simulink model "MOBATSim"  (R2020a)
settings: Solver=VariableStepAuto  StartTime=0.0  StopTime=20  FixedStep=0.01  RelTol=1e-3
undefined symbols (not defined in the file): default_spacing, FI_distance, FI_speed, max_ac, meters, min_ac, SafeDistance, Sim_Ts, simSpeed, time_gap, Ts, v_set, Vehicle1, Vehicle10, Vehicle2, Vehicle3, Vehicle4, Vehicle5, Vehicle6, Vehicle7, Vehicle8, Vehicle9, verr_gain, vx_gain, xerr_gain
libraries: simulink x32, mpcadaslib x1, robotalgslib x1
(part 2 of 4)

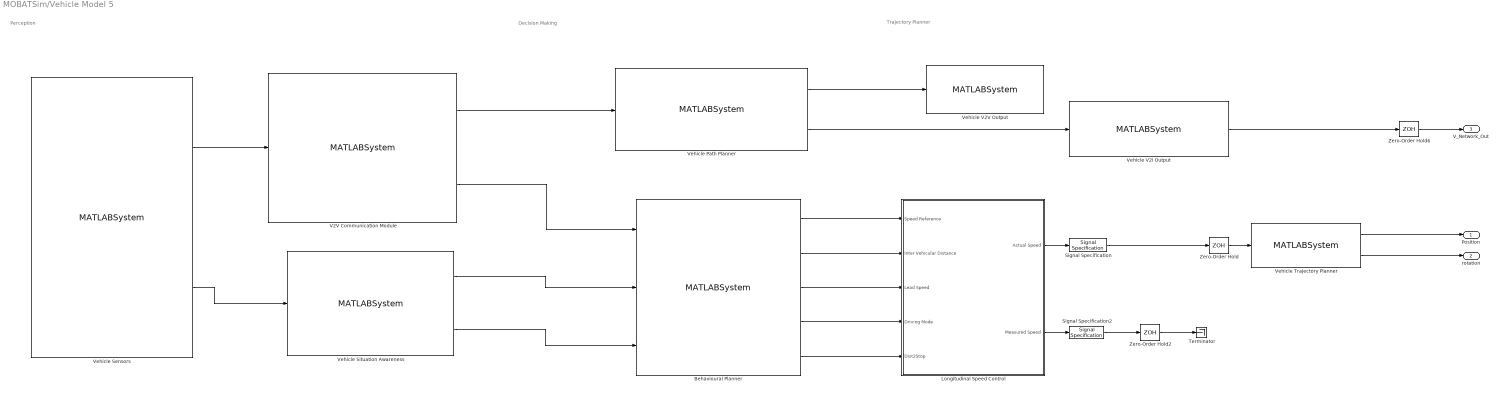
== system MOBATSim/Vehicle Model 5 ==
  note: Trajectory Planner
  note: Perception
  note: Decision Making
  Behavioural Planner : MATLABSystem  System=VehicleDrivingMode  Vehicle_id=Vehicle_id  SimulateUsing=Interpreted execution
      mask Type: VehicleDrivingMode
      mask Display:
      | image('BehaviouralPlanner.png');
      | port_label('input',1,'LeaderSpeed');
      | port_label('input',2,'LeaderDistance');
      | port_label('input',3,'emergencyCase');
      | port_label('output',1,'SpeedReference');
      | port_label('output',2,'DistanceReference');
      | port_label('output',3,'LeadSpeed');
      | port_label('output',4,'DrivingMode');
      | port_label('output',5,'Dist2Stop');
  Longitudinal Speed Control : Subsystem
  Signal Specification : SignalSpecification  Dimensions=1
  Signal Specification2 : SignalSpecification  Dimensions=1
  Terminator : Terminator
  V2V Communication Module : MATLABSystem  System=VehicleCommunication_v2v  Vehicle_id=Vehicle_id  SimulateUsing=Interpreted execution
      mask Type: VehicleCommunication_v2v
      mask Display:
      | image('V2V.png');
      | port_label('input',1,'CommunicationID');
      | port_label('output',1,'OtherVehiclesFutureData');
      | port_label('output',2,'LeaderSpeed');
  Vehicle Path Planner : MATLABSystem  System=VehiclePathPlanner  Vehicle_id=Vehicle_id  SimulateUsing=Interpreted execution
      mask Type: VehiclePathPlanner
      mask Display:
      | image('PathPlanner.png');
      | port_label('input',1,'OtherVehiclesFutureData');
      | port_label('output',1,'FuturePlan');
      | port_label('output',2,'waypointReached');
  Vehicle Sensors : MATLABSystem  System=VehicleSensors  Vehicle_id=Vehicle_id  Tsample=Sim_Ts  OffsetTime=0  SimulateUsing=Interpreted execution
      mask Type: VehicleSensors
      mask Display:
      | image('sensor.png');
      | port_label('output',1,'V2VcommIDs');
      | port_label('output',2,'ObjectinFront');
  Vehicle Situation Awareness : MATLABSystem  System=VehicleSituationAwareness  Vehicle_id=Vehicle_id  SimulateUsing=Interpreted execution
      mask Type: VehicleSituationAwareness
      mask Display:
      | image('situationAwareness.png');
      | port_label('input',1,'FrontSensorData');
      | port_label('output',1,'leaderDistance');
      | port_label('output',2,'emergencyCase');
  Vehicle Trajectory Planner : MATLABSystem  System=VehicleKinematics  Vehicle_id=Vehicle_id  SimulateUsing=Interpreted execution
      mask Type: VehicleKinematics
      mask Display:
      | image('Vehicle.png');
      | port_label('input',1,'speed');
      | port_label('output',1,'position');
      | port_label('output',2,'rotation');
  Vehicle V2I Output : MATLABSystem  System=VehicleV2I_Out  Vehicle_id=Vehicle_id  SimulateUsing=Interpreted execution
      mask Type: VehicleV2I_Out
      mask Display:
      | image('V2I.png');
      | port_label('input',1,'waypointReached');
      | port_label('output',1,'V2Idata');
  Vehicle V2V Output : MATLABSystem  System=VehicleNetwork_Out  Vehicle_id=Vehicle_id  SimulateUsing=Interpreted execution
      mask Type: VehicleNetwork_Out
      mask Display:
      | image('V2V.png');
      | port_label('input',1,'FuturePlan');
  Zero-Order Hold : ZeroOrderHold  SampleTime=Sim_Ts
  Zero-Order Hold2 : ZeroOrderHold  SampleTime=Sim_Ts
  Zero-Order Hold6 : ZeroOrderHold  SampleTime=Sim_Ts
  Position : Outport  VectorParamsAs1DForOutWhenUnconnected=off
  rotation : Outport  Port=2  VectorParamsAs1DForOutWhenUnconnected=off
  V_Network_Out : Outport  Port=3  VectorParamsAs1DForOutWhenUnconnected=off
  wires:
  Vehicle Trajectory Planner/1 -> Position/1
  Vehicle Trajectory Planner/2 -> rotation/1
  Signal Specification/1 -> Zero-Order Hold/1
  Zero-Order Hold/1 -> Vehicle Trajectory Planner/1
  Signal Specification2/1 -> Zero-Order Hold2/1
  Longitudinal Speed Control/1(Actual Speed) -> Signal Specification/1
  Vehicle V2I Output/1 -> Zero-Order Hold6/1
  Longitudinal Speed Control/2(Measured Speed) -> Signal Specification2/1
  Zero-Order Hold2/1 -> Terminator/1
  Vehicle Sensors/2 -> Vehicle Situation Awareness/1
  Vehicle Situation Awareness/2 -> Behavioural Planner/3
  Vehicle Situation Awareness/1 -> Behavioural Planner/2
  V2V Communication Module/2 -> Behavioural Planner/1
  V2V Communication Module/1 -> Vehicle Path Planner/1
  Behavioural Planner/5 -> Longitudinal Speed Control/5(Dist2Stop)
  Behavioural Planner/4 -> Longitudinal Speed Control/4(Driving Mode)
  Behavioural Planner/3 -> Longitudinal Speed Control/3(Lead Speed)
  Behavioural Planner/2 -> Longitudinal Speed Control/2(Inter Vehicular Distance)
  Behavioural Planner/1 -> Longitudinal Speed Control/1(Speed Reference)
  Vehicle Path Planner/2 -> Vehicle V2I Output/1
  Vehicle Path Planner/1 -> Vehicle V2V Output/1
  Vehicle Sensors/1 -> V2V Communication Module/1
  Zero-Order Hold6/1 -> V_Network_Out/1

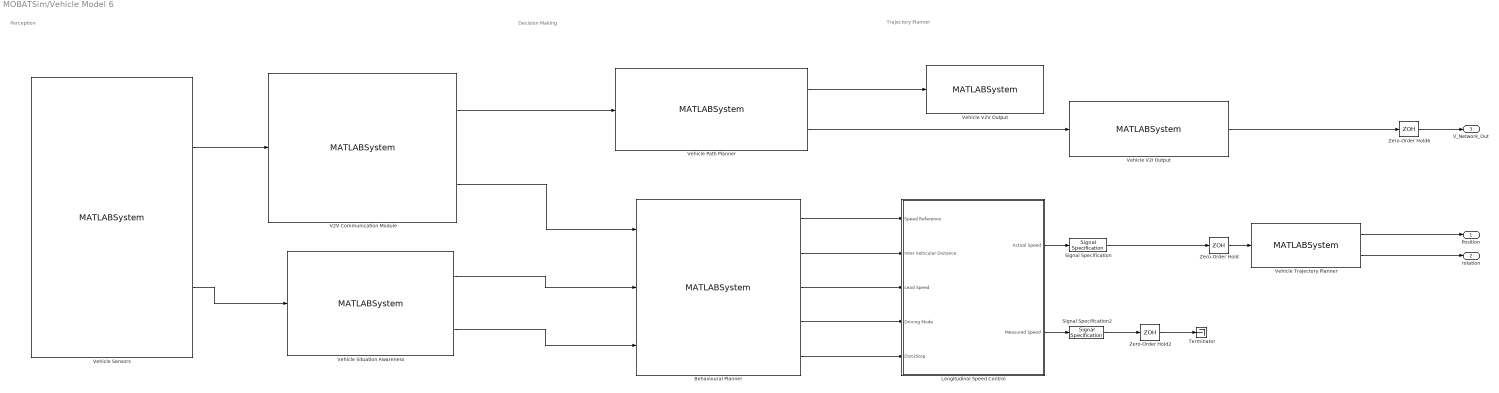
== system MOBATSim/Vehicle Model 6 ==
  note: Trajectory Planner
  note: Perception
  note: Decision Making
  Behavioural Planner : MATLABSystem  System=VehicleDrivingMode  Vehicle_id=Vehicle_id  SimulateUsing=Interpreted execution
      mask Type: VehicleDrivingMode
      mask Display:
      | image('BehaviouralPlanner.png');
      | port_label('input',1,'LeaderSpeed');
      | port_label('input',2,'LeaderDistance');
      | port_label('input',3,'emergencyCase');
      | port_label('output',1,'SpeedReference');
      | port_label('output',2,'DistanceReference');
      | port_label('output',3,'LeadSpeed');
      | port_label('output',4,'DrivingMode');
      | port_label('output',5,'Dist2Stop');
  Longitudinal Speed Control : Subsystem
  Signal Specification : SignalSpecification  Dimensions=1
  Signal Specification2 : SignalSpecification  Dimensions=1
  Terminator : Terminator
  V2V Communication Module : MATLABSystem  System=VehicleCommunication_v2v  Vehicle_id=Vehicle_id  SimulateUsing=Interpreted execution
      mask Type: VehicleCommunication_v2v
      mask Display:
      | image('V2V.png');
      | port_label('input',1,'CommunicationID');
      | port_label('output',1,'OtherVehiclesFutureData');
      | port_label('output',2,'LeaderSpeed');
  Vehicle Path Planner : MATLABSystem  System=VehiclePathPlanner  Vehicle_id=Vehicle_id  SimulateUsing=Interpreted execution
      mask Type: VehiclePathPlanner
      mask Display:
      | image('PathPlanner.png');
      | port_label('input',1,'OtherVehiclesFutureData');
      | port_label('output',1,'FuturePlan');
      | port_label('output',2,'waypointReached');
  Vehicle Sensors : MATLABSystem  System=VehicleSensors  Vehicle_id=Vehicle_id  Tsample=Sim_Ts  OffsetTime=0  SimulateUsing=Interpreted execution
      mask Type: VehicleSensors
      mask Display:
      | image('sensor.png');
      | port_label('output',1,'V2VcommIDs');
      | port_label('output',2,'ObjectinFront');
  Vehicle Situation Awareness : MATLABSystem  System=VehicleSituationAwareness  Vehicle_id=Vehicle_id  SimulateUsing=Interpreted execution
      mask Type: VehicleSituationAwareness
      mask Display:
      | image('situationAwareness.png');
      | port_label('input',1,'FrontSensorData');
      | port_label('output',1,'leaderDistance');
      | port_label('output',2,'emergencyCase');
  Vehicle Trajectory Planner : MATLABSystem  System=VehicleKinematics  Vehicle_id=Vehicle_id  SimulateUsing=Interpreted execution
      mask Type: VehicleKinematics
      mask Display:
      | image('Vehicle.png');
      | port_label('input',1,'speed');
      | port_label('output',1,'position');
      | port_label('output',2,'rotation');
  Vehicle V2I Output : MATLABSystem  System=VehicleV2I_Out  Vehicle_id=Vehicle_id  SimulateUsing=Interpreted execution
      mask Type: VehicleV2I_Out
      mask Display:
      | image('V2I.png');
      | port_label('input',1,'waypointReached');
      | port_label('output',1,'V2Idata');
  Vehicle V2V Output : MATLABSystem  System=VehicleNetwork_Out  Vehicle_id=Vehicle_id  SimulateUsing=Interpreted execution
      mask Type: VehicleNetwork_Out
      mask Display:
      | image('V2V.png');
      | port_label('input',1,'FuturePlan');
  Zero-Order Hold : ZeroOrderHold  SampleTime=Sim_Ts
  Zero-Order Hold2 : ZeroOrderHold  SampleTime=Sim_Ts
  Zero-Order Hold6 : ZeroOrderHold  SampleTime=Sim_Ts
  Position : Outport  VectorParamsAs1DForOutWhenUnconnected=off
  rotation : Outport  Port=2  VectorParamsAs1DForOutWhenUnconnected=off
  V_Network_Out : Outport  Port=3  VectorParamsAs1DForOutWhenUnconnected=off
  wires:
  Vehicle Trajectory Planner/1 -> Position/1
  Vehicle Trajectory Planner/2 -> rotation/1
  Signal Specification/1 -> Zero-Order Hold/1
  Zero-Order Hold/1 -> Vehicle Trajectory Planner/1
  Signal Specification2/1 -> Zero-Order Hold2/1
  Longitudinal Speed Control/1(Actual Speed) -> Signal Specification/1
  Vehicle V2I Output/1 -> Zero-Order Hold6/1
  Longitudinal Speed Control/2(Measured Speed) -> Signal Specification2/1
  Zero-Order Hold2/1 -> Terminator/1
  Vehicle Sensors/2 -> Vehicle Situation Awareness/1
  Vehicle Situation Awareness/2 -> Behavioural Planner/3
  Vehicle Situation Awareness/1 -> Behavioural Planner/2
  V2V Communication Module/2 -> Behavioural Planner/1
  V2V Communication Module/1 -> Vehicle Path Planner/1
  Behavioural Planner/5 -> Longitudinal Speed Control/5(Dist2Stop)
  Behavioural Planner/4 -> Longitudinal Speed Control/4(Driving Mode)
  Behavioural Planner/3 -> Longitudinal Speed Control/3(Lead Speed)
  Behavioural Planner/2 -> Longitudinal Speed Control/2(Inter Vehicular Distance)
  Behavioural Planner/1 -> Longitudinal Speed Control/1(Speed Reference)
  Vehicle Path Planner/2 -> Vehicle V2I Output/1
  Vehicle Path Planner/1 -> Vehicle V2V Output/1
  Vehicle Sensors/1 -> V2V Communication Module/1
  Zero-Order Hold6/1 -> V_Network_Out/1

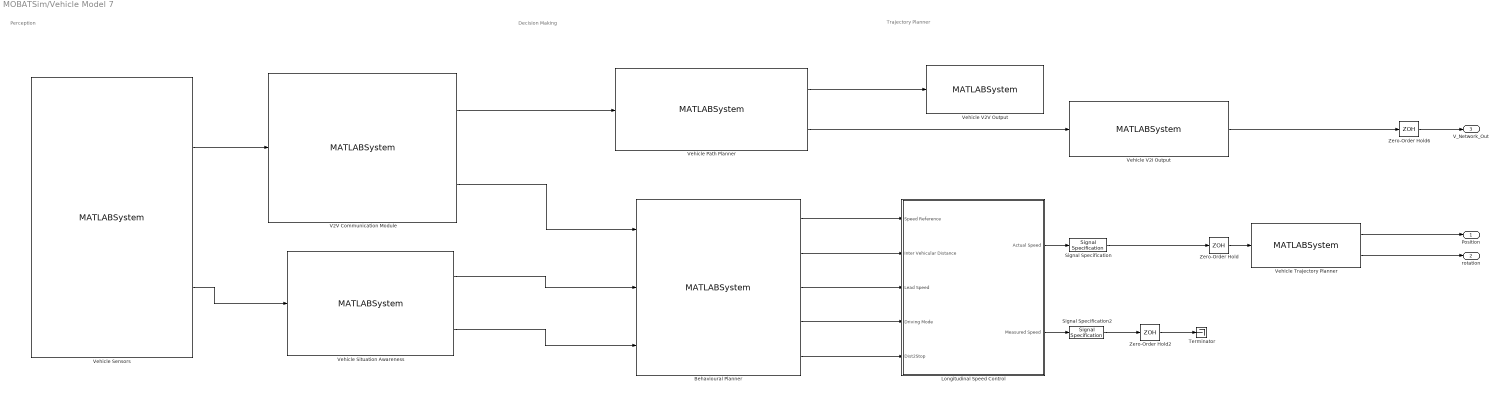
== system MOBATSim/Vehicle Model 7 ==
  note: Trajectory Planner
  note: Perception
  note: Decision Making
  Behavioural Planner : MATLABSystem  System=VehicleDrivingMode  Vehicle_id=Vehicle_id  SimulateUsing=Interpreted execution
      mask Type: VehicleDrivingMode
      mask Display:
      | image('BehaviouralPlanner.png');
      | port_label('input',1,'LeaderSpeed');
      | port_label('input',2,'LeaderDistance');
      | port_label('input',3,'emergencyCase');
      | port_label('output',1,'SpeedReference');
      | port_label('output',2,'DistanceReference');
      | port_label('output',3,'LeadSpeed');
      | port_label('output',4,'DrivingMode');
      | port_label('output',5,'Dist2Stop');
  Longitudinal Speed Control : Subsystem
  Signal Specification : SignalSpecification  Dimensions=1
  Signal Specification2 : SignalSpecification  Dimensions=1
  Terminator : Terminator
  V2V Communication Module : MATLABSystem  System=VehicleCommunication_v2v  Vehicle_id=Vehicle_id  SimulateUsing=Interpreted execution
      mask Type: VehicleCommunication_v2v
      mask Display:
      | image('V2V.png');
      | port_label('input',1,'CommunicationID');
      | port_label('output',1,'OtherVehiclesFutureData');
      | port_label('output',2,'LeaderSpeed');
  Vehicle Path Planner : MATLABSystem  System=VehiclePathPlanner  Vehicle_id=Vehicle_id  SimulateUsing=Interpreted execution
      mask Type: VehiclePathPlanner
      mask Display:
      | image('PathPlanner.png');
      | port_label('input',1,'OtherVehiclesFutureData');
      | port_label('output',1,'FuturePlan');
      | port_label('output',2,'waypointReached');
  Vehicle Sensors : MATLABSystem  System=VehicleSensors  Vehicle_id=Vehicle_id  Tsample=Sim_Ts  OffsetTime=0  SimulateUsing=Interpreted execution
      mask Type: VehicleSensors
      mask Display:
      | image('sensor.png');
      | port_label('output',1,'V2VcommIDs');
      | port_label('output',2,'ObjectinFront');
  Vehicle Situation Awareness : MATLABSystem  System=VehicleSituationAwareness  Vehicle_id=Vehicle_id  SimulateUsing=Interpreted execution
      mask Type: VehicleSituationAwareness
      mask Display:
      | image('situationAwareness.png');
      | port_label('input',1,'FrontSensorData');
      | port_label('output',1,'leaderDistance');
      | port_label('output',2,'emergencyCase');
  Vehicle Trajectory Planner : MATLABSystem  System=VehicleKinematics  Vehicle_id=Vehicle_id  SimulateUsing=Interpreted execution
      mask Type: VehicleKinematics
      mask Display:
      | image('Vehicle.png');
      | port_label('input',1,'speed');
      | port_label('output',1,'position');
      | port_label('output',2,'rotation');
  Vehicle V2I Output : MATLABSystem  System=VehicleV2I_Out  Vehicle_id=Vehicle_id  SimulateUsing=Interpreted execution
      mask Type: VehicleV2I_Out
      mask Display:
      | image('V2I.png');
      | port_label('input',1,'waypointReached');
      | port_label('output',1,'V2Idata');
  Vehicle V2V Output : MATLABSystem  System=VehicleNetwork_Out  Vehicle_id=Vehicle_id  SimulateUsing=Interpreted execution
      mask Type: VehicleNetwork_Out
      mask Display:
      | image('V2V.png');
      | port_label('input',1,'FuturePlan');
  Zero-Order Hold : ZeroOrderHold  SampleTime=Sim_Ts
  Zero-Order Hold2 : ZeroOrderHold  SampleTime=Sim_Ts
  Zero-Order Hold6 : ZeroOrderHold  SampleTime=Sim_Ts
  Position : Outport  VectorParamsAs1DForOutWhenUnconnected=off
  rotation : Outport  Port=2  VectorParamsAs1DForOutWhenUnconnected=off
  V_Network_Out : Outport  Port=3  VectorParamsAs1DForOutWhenUnconnected=off
  wires:
  Vehicle Trajectory Planner/1 -> Position/1
  Vehicle Trajectory Planner/2 -> rotation/1
  Signal Specification/1 -> Zero-Order Hold/1
  Zero-Order Hold/1 -> Vehicle Trajectory Planner/1
  Signal Specification2/1 -> Zero-Order Hold2/1
  Longitudinal Speed Control/1(Actual Speed) -> Signal Specification/1
  Vehicle V2I Output/1 -> Zero-Order Hold6/1
  Longitudinal Speed Control/2(Measured Speed) -> Signal Specification2/1
  Zero-Order Hold2/1 -> Terminator/1
  Vehicle Sensors/2 -> Vehicle Situation Awareness/1
  Vehicle Situation Awareness/2 -> Behavioural Planner/3
  Vehicle Situation Awareness/1 -> Behavioural Planner/2
  V2V Communication Module/2 -> Behavioural Planner/1
  V2V Communication Module/1 -> Vehicle Path Planner/1
  Behavioural Planner/5 -> Longitudinal Speed Control/5(Dist2Stop)
  Behavioural Planner/4 -> Longitudinal Speed Control/4(Driving Mode)
  Behavioural Planner/3 -> Longitudinal Speed Control/3(Lead Speed)
  Behavioural Planner/2 -> Longitudinal Speed Control/2(Inter Vehicular Distance)
  Behavioural Planner/1 -> Longitudinal Speed Control/1(Speed Reference)
  Vehicle Path Planner/2 -> Vehicle V2I Output/1
  Vehicle Path Planner/1 -> Vehicle V2V Output/1
  Vehicle Sensors/1 -> V2V Communication Module/1
  Zero-Order Hold6/1 -> V_Network_Out/1

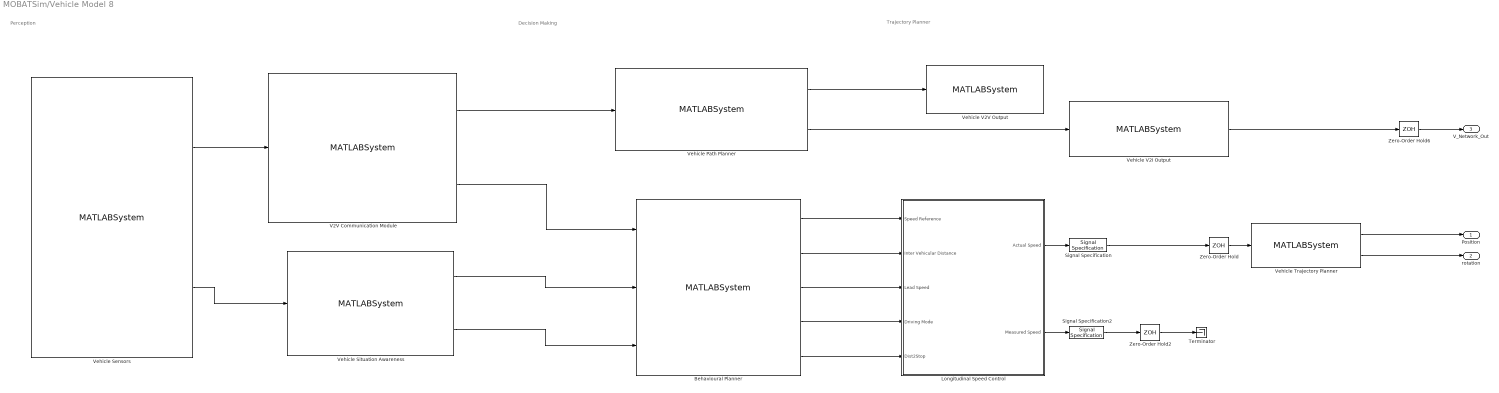
== system MOBATSim/Vehicle Model 8 ==
  note: Trajectory Planner
  note: Perception
  note: Decision Making
  Behavioural Planner : MATLABSystem  System=VehicleDrivingMode  Vehicle_id=Vehicle_id  SimulateUsing=Interpreted execution
      mask Type: VehicleDrivingMode
      mask Display:
      | image('BehaviouralPlanner.png');
      | port_label('input',1,'LeaderSpeed');
      | port_label('input',2,'LeaderDistance');
      | port_label('input',3,'emergencyCase');
      | port_label('output',1,'SpeedReference');
      | port_label('output',2,'DistanceReference');
      | port_label('output',3,'LeadSpeed');
      | port_label('output',4,'DrivingMode');
      | port_label('output',5,'Dist2Stop');
  Longitudinal Speed Control : Subsystem
  Signal Specification : SignalSpecification  Dimensions=1
  Signal Specification2 : SignalSpecification  Dimensions=1
  Terminator : Terminator
  V2V Communication Module : MATLABSystem  System=VehicleCommunication_v2v  Vehicle_id=Vehicle_id  SimulateUsing=Interpreted execution
      mask Type: VehicleCommunication_v2v
      mask Display:
      | image('V2V.png');
      | port_label('input',1,'CommunicationID');
      | port_label('output',1,'OtherVehiclesFutureData');
      | port_label('output',2,'LeaderSpeed');
  Vehicle Path Planner : MATLABSystem  System=VehiclePathPlanner  Vehicle_id=Vehicle_id  SimulateUsing=Interpreted execution
      mask Type: VehiclePathPlanner
      mask Display:
      | image('PathPlanner.png');
      | port_label('input',1,'OtherVehiclesFutureData');
      | port_label('output',1,'FuturePlan');
      | port_label('output',2,'waypointReached');
  Vehicle Sensors : MATLABSystem  System=VehicleSensors  Vehicle_id=Vehicle_id  Tsample=Sim_Ts  OffsetTime=0  SimulateUsing=Interpreted execution
      mask Type: VehicleSensors
      mask Display:
      | image('sensor.png');
      | port_label('output',1,'V2VcommIDs');
      | port_label('output',2,'ObjectinFront');
  Vehicle Situation Awareness : MATLABSystem  System=VehicleSituationAwareness  Vehicle_id=Vehicle_id  SimulateUsing=Interpreted execution
      mask Type: VehicleSituationAwareness
      mask Display:
      | image('situationAwareness.png');
      | port_label('input',1,'FrontSensorData');
      | port_label('output',1,'leaderDistance');
      | port_label('output',2,'emergencyCase');
  Vehicle Trajectory Planner : MATLABSystem  System=VehicleKinematics  Vehicle_id=Vehicle_id  SimulateUsing=Interpreted execution
      mask Type: VehicleKinematics
      mask Display:
      | image('Vehicle.png');
      | port_label('input',1,'speed');
      | port_label('output',1,'position');
      | port_label('output',2,'rotation');
  Vehicle V2I Output : MATLABSystem  System=VehicleV2I_Out  Vehicle_id=Vehicle_id  SimulateUsing=Interpreted execution
      mask Type: VehicleV2I_Out
      mask Display:
      | image('V2I.png');
      | port_label('input',1,'waypointReached');
      | port_label('output',1,'V2Idata');
  Vehicle V2V Output : MATLABSystem  System=VehicleNetwork_Out  Vehicle_id=Vehicle_id  SimulateUsing=Interpreted execution
      mask Type: VehicleNetwork_Out
      mask Display:
      | image('V2V.png');
      | port_label('input',1,'FuturePlan');
  Zero-Order Hold : ZeroOrderHold  SampleTime=Sim_Ts
  Zero-Order Hold2 : ZeroOrderHold  SampleTime=Sim_Ts
  Zero-Order Hold6 : ZeroOrderHold  SampleTime=Sim_Ts
  Position : Outport  VectorParamsAs1DForOutWhenUnconnected=off
  rotation : Outport  Port=2  VectorParamsAs1DForOutWhenUnconnected=off
  V_Network_Out : Outport  Port=3  VectorParamsAs1DForOutWhenUnconnected=off
  wires:
  Vehicle Trajectory Planner/1 -> Position/1
  Vehicle Trajectory Planner/2 -> rotation/1
  Signal Specification/1 -> Zero-Order Hold/1
  Zero-Order Hold/1 -> Vehicle Trajectory Planner/1
  Signal Specification2/1 -> Zero-Order Hold2/1
  Longitudinal Speed Control/1(Actual Speed) -> Signal Specification/1
  Vehicle V2I Output/1 -> Zero-Order Hold6/1
  Longitudinal Speed Control/2(Measured Speed) -> Signal Specification2/1
  Zero-Order Hold2/1 -> Terminator/1
  Vehicle Sensors/2 -> Vehicle Situation Awareness/1
  Vehicle Situation Awareness/2 -> Behavioural Planner/3
  Vehicle Situation Awareness/1 -> Behavioural Planner/2
  V2V Communication Module/2 -> Behavioural Planner/1
  V2V Communication Module/1 -> Vehicle Path Planner/1
  Behavioural Planner/5 -> Longitudinal Speed Control/5(Dist2Stop)
  Behavioural Planner/4 -> Longitudinal Speed Control/4(Driving Mode)
  Behavioural Planner/3 -> Longitudinal Speed Control/3(Lead Speed)
  Behavioural Planner/2 -> Longitudinal Speed Control/2(Inter Vehicular Distance)
  Behavioural Planner/1 -> Longitudinal Speed Control/1(Speed Reference)
  Vehicle Path Planner/2 -> Vehicle V2I Output/1
  Vehicle Path Planner/1 -> Vehicle V2V Output/1
  Vehicle Sensors/1 -> V2V Communication Module/1
  Zero-Order Hold6/1 -> V_Network_Out/1

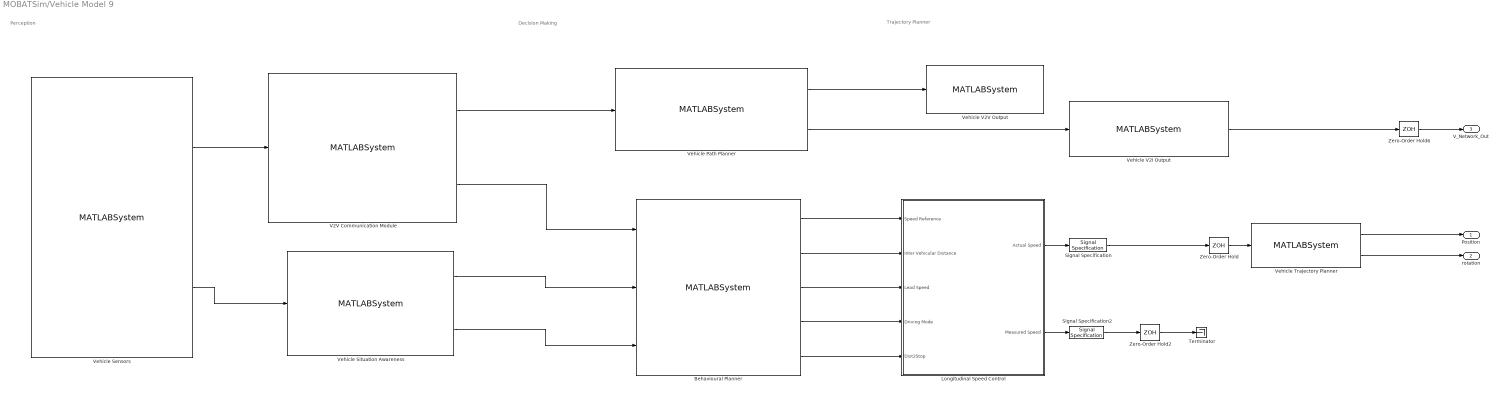
== system MOBATSim/Vehicle Model 9 ==
  note: Trajectory Planner
  note: Perception
  note: Decision Making
  Behavioural Planner : MATLABSystem  System=VehicleDrivingMode  Vehicle_id=Vehicle_id  SimulateUsing=Interpreted execution
      mask Type: VehicleDrivingMode
      mask Display:
      | image('BehaviouralPlanner.png');
      | port_label('input',1,'LeaderSpeed');
      | port_label('input',2,'LeaderDistance');
      | port_label('input',3,'emergencyCase');
      | port_label('output',1,'SpeedReference');
      | port_label('output',2,'DistanceReference');
      | port_label('output',3,'LeadSpeed');
      | port_label('output',4,'DrivingMode');
      | port_label('output',5,'Dist2Stop');
  Longitudinal Speed Control : Subsystem
  Signal Specification : SignalSpecification  Dimensions=1
  Signal Specification2 : SignalSpecification  Dimensions=1
  Terminator : Terminator
  V2V Communication Module : MATLABSystem  System=VehicleCommunication_v2v  Vehicle_id=Vehicle_id  SimulateUsing=Interpreted execution
      mask Type: VehicleCommunication_v2v
      mask Display:
      | image('V2V.png');
      | port_label('input',1,'CommunicationID');
      | port_label('output',1,'OtherVehiclesFutureData');
      | port_label('output',2,'LeaderSpeed');
  Vehicle Path Planner : MATLABSystem  System=VehiclePathPlanner  Vehicle_id=Vehicle_id  SimulateUsing=Interpreted execution
      mask Type: VehiclePathPlanner
      mask Display:
      | image('PathPlanner.png');
      | port_label('input',1,'OtherVehiclesFutureData');
      | port_label('output',1,'FuturePlan');
      | port_label('output',2,'waypointReached');
  Vehicle Sensors : MATLABSystem  System=VehicleSensors  Vehicle_id=Vehicle_id  Tsample=Sim_Ts  OffsetTime=0  SimulateUsing=Interpreted execution
      mask Type: VehicleSensors
      mask Display:
      | image('sensor.png');
      | port_label('output',1,'V2VcommIDs');
      | port_label('output',2,'ObjectinFront');
  Vehicle Situation Awareness : MATLABSystem  System=VehicleSituationAwareness  Vehicle_id=Vehicle_id  SimulateUsing=Interpreted execution
      mask Type: VehicleSituationAwareness
      mask Display:
      | image('situationAwareness.png');
      | port_label('input',1,'FrontSensorData');
      | port_label('output',1,'leaderDistance');
      | port_label('output',2,'emergencyCase');
  Vehicle Trajectory Planner : MATLABSystem  System=VehicleKinematics  Vehicle_id=Vehicle_id  SimulateUsing=Interpreted execution
      mask Type: VehicleKinematics
      mask Display:
      | image('Vehicle.png');
      | port_label('input',1,'speed');
      | port_label('output',1,'position');
      | port_label('output',2,'rotation');
  Vehicle V2I Output : MATLABSystem  System=VehicleV2I_Out  Vehicle_id=Vehicle_id  SimulateUsing=Interpreted execution
      mask Type: VehicleV2I_Out
      mask Display:
      | image('V2I.png');
      | port_label('input',1,'waypointReached');
      | port_label('output',1,'V2Idata');
  Vehicle V2V Output : MATLABSystem  System=VehicleNetwork_Out  Vehicle_id=Vehicle_id  SimulateUsing=Interpreted execution
      mask Type: VehicleNetwork_Out
      mask Display:
      | image('V2V.png');
      | port_label('input',1,'FuturePlan');
  Zero-Order Hold : ZeroOrderHold  SampleTime=Sim_Ts
  Zero-Order Hold2 : ZeroOrderHold  SampleTime=Sim_Ts
  Zero-Order Hold6 : ZeroOrderHold  SampleTime=Sim_Ts
  Position : Outport  VectorParamsAs1DForOutWhenUnconnected=off
  rotation : Outport  Port=2  VectorParamsAs1DForOutWhenUnconnected=off
  V_Network_Out : Outport  Port=3  VectorParamsAs1DForOutWhenUnconnected=off
  wires:
  Vehicle Trajectory Planner/1 -> Position/1
  Vehicle Trajectory Planner/2 -> rotation/1
  Signal Specification/1 -> Zero-Order Hold/1
  Zero-Order Hold/1 -> Vehicle Trajectory Planner/1
  Signal Specification2/1 -> Zero-Order Hold2/1
  Longitudinal Speed Control/1(Actual Speed) -> Signal Specification/1
  Vehicle V2I Output/1 -> Zero-Order Hold6/1
  Longitudinal Speed Control/2(Measured Speed) -> Signal Specification2/1
  Zero-Order Hold2/1 -> Terminator/1
  Vehicle Sensors/2 -> Vehicle Situation Awareness/1
  Vehicle Situation Awareness/2 -> Behavioural Planner/3
  Vehicle Situation Awareness/1 -> Behavioural Planner/2
  V2V Communication Module/2 -> Behavioural Planner/1
  V2V Communication Module/1 -> Vehicle Path Planner/1
  Behavioural Planner/5 -> Longitudinal Speed Control/5(Dist2Stop)
  Behavioural Planner/4 -> Longitudinal Speed Control/4(Driving Mode)
  Behavioural Planner/3 -> Longitudinal Speed Control/3(Lead Speed)
  Behavioural Planner/2 -> Longitudinal Speed Control/2(Inter Vehicular Distance)
  Behavioural Planner/1 -> Longitudinal Speed Control/1(Speed Reference)
  Vehicle Path Planner/2 -> Vehicle V2I Output/1
  Vehicle Path Planner/1 -> Vehicle V2V Output/1
  Vehicle Sensors/1 -> V2V Communication Module/1
  Zero-Order Hold6/1 -> V_Network_Out/1

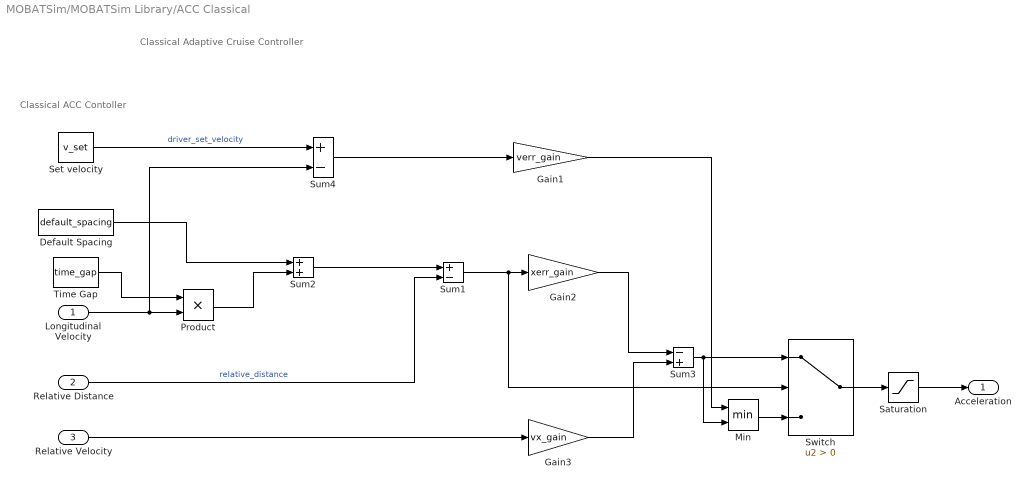
== system MOBATSim/MOBATSim Library/ACC Classical ==
  note: Classical ACC Contoller
  note: Classical Adaptive Cruise Controller
  Longitudinal Velocity : Inport
  Relative Distance : Inport  Port=2
  Relative Velocity : Inport  Port=3
  Default Spacing : Constant  Value=default_spacing  SampleTime=Ts
  Gain1 : Gain  Gain=verr_gain
  Gain2 : Gain  Gain=xerr_gain
  Gain3 : Gain  Gain=vx_gain
  Min : MinMax  Inputs=2
  Product : Product
  Saturation : Saturate  UpperLimit=max_ac  LowerLimit=min_ac
  Set velocity : Constant  Value=v_set  SampleTime=Ts
  Sum1 : Sum  Inputs=+-
  Sum2 : Sum
  Sum3 : Sum  Inputs=-+
  Sum4 : Sum  Inputs=+-
  Switch : Switch  Criteria=u2 > Threshold
  Time Gap : Constant  Value=time_gap  SampleTime=Ts
  Acceleration : Outport  VectorParamsAs1DForOutWhenUnconnected=off
  wires:
  Longitudinal Velocity/1 -> Product/2, Sum4/2
  Default Spacing/1 -> Sum2/1
  Gain2/1 -> Sum3/1
  Sum4/1 -> Gain1/1
  Min/1 -> Switch/3
  Gain3/1 -> Sum3/2
  Switch/1 -> Saturation/1
  Relative Velocity/1 -> Gain3/1
  Time Gap/1 -> Product/1
  Saturation/1 -> Acceleration/1
  Product/1 -> Sum2/2
  Set velocity/1 -> Sum4/1  "driver_set_velocity"
  Sum3/1 -> Min/2, Switch/1
  Sum1/1 -> Switch/2, Gain2/1
  Gain1/1 -> Min/1
  Relative Distance/1 -> Sum1/2  "relative_distance"
  Sum2/1 -> Sum1/1

== system MOBATSim/MOBATSim Library/Platoon Controller - PID ==
  Inter Vehicular Distance : Inport
  Lead Speed : Inport  Port=2
  Vehicle Speed : Inport  Port=3
  Compare To Constant : simulink/Logic and Bit Operations/Compare To Constant  relop=>  const=2  OutDataTypeStr=uint8
  Constant : Constant  Value=meters
  Gain : Gain  Gain=1.4
  Multiport Switch : MultiPortSwitch  DataPortOrder=Zero-based contiguous  Inputs=2  zeroidx=on
  PID Controller5 : simulink/Continuous/PID Controller  Controller=PID  Form=Parallel  TimeDomain=Continuous-time  UseExternalTs=off  SampleTime=-1  IntegratorMethod=Forward Euler  FilterMethod=Forward Euler  ControllerParametersSource=internal  P=2.0341199375219  I=0.0356576460366845  D=2.08363010404189  UseFilter=on  N=233.214579742572  TunerSelectOption=Transfer Function Based (PID Tuner App)  InitialConditionSource=internal  InitialConditionForIntegrator=0  InitialConditionForFilter=0  DifferentiatorICPrevScaledInput=0  ExternalReset=none  TrackingMode=off  Kt=1  LimitOutput=on  UpperSaturationLimit=100  LowerSaturationLimit=-100  LinearizeAsGain=on  AntiWindupMode=clamping  Kb=1  POutMin=[]  POutMax=[]  IOutMin=[]  IOutMax=[]  DOutMin=[]  DOutMax=[]  NOutMin=[]  NOutMax=[]  SumOutMin=[]  SumOutMax=[]  SaturationOutMin=[]  SaturationOutMax=[]  PParamMin=[]  PParamMax=[]  IParamMin=[]  IParamMax=[]  DParamMin=[]  DParamMax=[]  NParamMin=[]  NParamMax=[]  KbParamMin=[]  KbParamMax=[]  KtParamMin=[]  KtParamMax=[]  KbOutMin=[]  KbOutMax=[]  KtOutMin=[]  KtOutMax=[]  IntegratorOutMin=[]  IntegratorOutMax=[]  FilterOutMin=[]  FilterOutMax=[]  SumI1OutMin=[]  SumI1OutMax=[]  SumI2OutMin=[]  SumI2OutMax=[]  SumI3OutMin=[]  SumI3OutMax=[]  SumI4OutMin=[]  SumI4OutMax=[]  SumDOutMin=[]  SumDOutMax=[]  DifferentiatorOutMin=[]  DifferentiatorOutMax=[]  FilterDiffOutCoefMin=[]  FilterDiffOutCoefMax=[]  ReciprocalOutMin=[]  ReciprocalOutMax=[]  SumDenOutMin=[]  SumDenOutMax=[]  SumNumOutMin=[]  SumNumOutMax=[]  DivideOutMin=[]  DivideOutMax=[]  UdiffTsProdOutMin=[]  UdiffTsProdOutMax=[]  NTsProdOutMin=[]  NTsProdOutMax=[]  UintegralTsProdOutMin=[]  UintegralTsProdOutMax=[]  UngainTsProdOutMin=[]  UngainTsProdOutMax=[]  IntegratorContinuousStateAttributes=''  IntegratorStateMustResolveToSignalObject=off  IntegratorRTWStateStorageClass=Auto  FilterContinuousStateAttributes=''  FilterStateMustResolveToSignalObject=off  FilterRTWStateStorageClass=Auto  ParallelPVariant=InternalParameters  IdealPVariant=Disabled  IVariant=InternalParameters  DVariant=InternalParameters  IntegratorVariant=Continuous  SatVariant=Enabled  AWVariant=ContClampingParallel  PCopyVariant=Disabled  TRVariant=Disabled  FdbkBlocksVariant=Forward  IdealPFdbkVariant=Disabled  SatFdbkVariant=Disabled  DerivativeFilterVariant=ContFilter  NVariant=InternalParameters  NCopyVariant=Disabled  FilterICVariant=InternalICsFilter  IntegratorICVariant=InternalICs  ExternalResetVariant=Disabled  TRSumVariant=Passthrough  SumFdbkVariant=Disabled  SumVariant=Sum_PID  TsampFilterVariant=InternalTs  TsampNgainVariant=Passthrough  TsampIntegralVariant=Passthrough
  Sum : Sum  Inputs=|-+
  Sum1 : Sum  Inputs=|++
  Sum2 : Sum  Inputs=|+-
  Transfer Fcn : TransferFcn  Numerator=[0.05]  Denominator=[1 2]
  ref speed : Outport  VectorParamsAs1DForOutWhenUnconnected=off
  wires:
  Transfer Fcn/1 -> PID Controller5/1
  Vehicle Speed/1 -> Gain/1, Sum/1
  PID Controller5/1 -> Multiport Switch/2
  Sum/1 -> Compare To Constant/1
  Multiport Switch/1 -> ref speed/1
  Compare To Constant/1 -> Multiport Switch/1
  Lead Speed/1 -> Sum/2, Multiport Switch/3
  Constant/1 -> Sum1/1
  Sum1/1 -> Sum2/2
  Gain/1 -> Sum1/2
  Sum2/1 -> Transfer Fcn/1
  Inter Vehicular Distance/1 -> Sum2/1

== system MOBATSim/Vehicle Model 1/Longitudinal Speed Control ==
  note: Here the measured speed and the actual speed are the same
      | but it is designed to include the effects of the measurement errors
  note: The vehicle calculates the speed difference between the actual speed and the reference speed, then generates the acceleration command accordingly.
  Speed Reference : Inport
  Inter Vehicular Distance : Inport  Port=2
  Lead Speed : Inport  Port=3
  Driving Mode : Inport  Port=4
  Dist2Stop : Inport  Port=5
  Acceleration Command : Subsystem
  Distance to Stop Controller : Subsystem
  Platoon Controller : Subsystem
  Reference speed according to the driving mode : Subsystem
  Signal Specification1 : SignalSpecification  Dimensions=1
  Sum13 : Sum  Inputs=|+-
  Vehicle Dynamic Model : Subsystem
  Actual Speed : Outport  VectorParamsAs1DForOutWhenUnconnected=off
  Measured Speed : Outport  Port=2  VectorParamsAs1DForOutWhenUnconnected=off
  wires:
  Platoon Controller/1(ref speed) -> Distance to Stop Controller/1(Speed Ref from Platoon), Reference speed according to the driving mode/3(In3)
  Lead Speed/1 -> Platoon Controller/2(Lead Speed)
  Driving Mode/1 -> Acceleration Command/1(Driving Mode), Reference speed according to the driving mode/1(In1)
  Signal Specification1/1 -> Actual Speed/1
  Sum13/1 -> Acceleration Command/2(Speed Error)
  Inter Vehicular Distance/1 -> Platoon Controller/1(Inter Vehicular Distance)
  Dist2Stop/1 -> Distance to Stop Controller/2(Distance to Stop)
  Speed Reference/1 -> Reference speed according to the driving mode/2(In2)
  Distance to Stop Controller/1(ref speed) -> Reference speed according to the driving mode/4(In4)
  Reference speed according to the driving mode/1(Out1) -> Sum13/1
  Vehicle Dynamic Model/1(Vehicle Speed) -> Signal Specification1/1, Acceleration Command/3(Actual Speed), Sum13/2, Platoon Controller/3(Vehicle Speed), Measured Speed/1
  Acceleration Command/1(Acceleration Command) -> Vehicle Dynamic Model/1(Acceleration Command)

== system MOBATSim/Vehicle Model 10/Longitudinal Speed Control ==
  note: Here the measured speed and the actual speed are the same
      | but it is designed to include the effects of the measurement errors
  note: The vehicle calculates the speed difference between the actual speed and the reference speed, then generates the acceleration command accordingly.
  Speed Reference : Inport
  Inter Vehicular Distance : Inport  Port=2
  Lead Speed : Inport  Port=3
  Driving Mode : Inport  Port=4
  Dist2Stop : Inport  Port=5
  Acceleration Command : Subsystem
  Distance to Stop Controller : Subsystem
  Platoon Controller : Subsystem
  Reference speed according to the driving mode : Subsystem
  Signal Specification1 : SignalSpecification  Dimensions=1
  Sum13 : Sum  Inputs=|+-
  Vehicle Dynamic Model : Subsystem
  Actual Speed : Outport  VectorParamsAs1DForOutWhenUnconnected=off
  Measured Speed : Outport  Port=2  VectorParamsAs1DForOutWhenUnconnected=off
  wires:
  Platoon Controller/1(ref speed) -> Distance to Stop Controller/1(Speed Ref from Platoon), Reference speed according to the driving mode/3(In3)
  Lead Speed/1 -> Platoon Controller/2(Lead Speed)
  Driving Mode/1 -> Acceleration Command/1(Driving Mode), Reference speed according to the driving mode/1(In1)
  Signal Specification1/1 -> Actual Speed/1
  Sum13/1 -> Acceleration Command/2(Speed Error)
  Inter Vehicular Distance/1 -> Platoon Controller/1(Inter Vehicular Distance)
  Dist2Stop/1 -> Distance to Stop Controller/2(Distance to Stop)
  Speed Reference/1 -> Reference speed according to the driving mode/2(In2)
  Distance to Stop Controller/1(ref speed) -> Reference speed according to the driving mode/4(In4)
  Reference speed according to the driving mode/1(Out1) -> Sum13/1
  Vehicle Dynamic Model/1(Vehicle Speed) -> Signal Specification1/1, Acceleration Command/3(Actual Speed), Sum13/2, Platoon Controller/3(Vehicle Speed), Measured Speed/1
  Acceleration Command/1(Acceleration Command) -> Vehicle Dynamic Model/1(Acceleration Command)

== system MOBATSim/Vehicle Model 2/Longitudinal Speed Control ==
  note: Here the measured speed and the actual speed are the same
      | but it is designed to include the effects of the measurement errors
  note: The vehicle calculates the speed difference between the actual speed and the reference speed, then generates the acceleration command accordingly.
  Speed Reference : Inport
  Inter Vehicular Distance : Inport  Port=2
  Lead Speed : Inport  Port=3
  Driving Mode : Inport  Port=4
  Dist2Stop : Inport  Port=5
  Acceleration Command : Subsystem
  Distance to Stop Controller : Subsystem
  Platoon Controller : Subsystem
  Reference speed according to the driving mode : Subsystem
  Signal Specification1 : SignalSpecification  Dimensions=1
  Sum13 : Sum  Inputs=|+-
  Vehicle Dynamic Model : Subsystem
  Actual Speed : Outport  VectorParamsAs1DForOutWhenUnconnected=off
  Measured Speed : Outport  Port=2  VectorParamsAs1DForOutWhenUnconnected=off
  wires:
  Platoon Controller/1(ref speed) -> Distance to Stop Controller/1(Speed Ref from Platoon), Reference speed according to the driving mode/3(In3)
  Lead Speed/1 -> Platoon Controller/2(Lead Speed)
  Driving Mode/1 -> Acceleration Command/1(Driving Mode), Reference speed according to the driving mode/1(In1)
  Signal Specification1/1 -> Actual Speed/1
  Sum13/1 -> Acceleration Command/2(Speed Error)
  Inter Vehicular Distance/1 -> Platoon Controller/1(Inter Vehicular Distance)
  Dist2Stop/1 -> Distance to Stop Controller/2(Distance to Stop)
  Speed Reference/1 -> Reference speed according to the driving mode/2(In2)
  Distance to Stop Controller/1(ref speed) -> Reference speed according to the driving mode/4(In4)
  Reference speed according to the driving mode/1(Out1) -> Sum13/1
  Vehicle Dynamic Model/1(Vehicle Speed) -> Signal Specification1/1, Acceleration Command/3(Actual Speed), Sum13/2, Platoon Controller/3(Vehicle Speed), Measured Speed/1
  Acceleration Command/1(Acceleration Command) -> Vehicle Dynamic Model/1(Acceleration Command)

== system MOBATSim/Vehicle Model 2/TransitionMatrix ==
  In1 : Inport
  In2 : Inport  Port=2
  Constant : Constant  Value=1.5*pi
  Gain1 : Gain  Gain=-1
  Mux1 : Mux  Inputs=3
  Selector : Selector  InputPortWidth=3  IndexOptions=Index vector (dialog)  Indices=[1]  OutputSizes=1
  Selector1 : Selector  InputPortWidth=3  IndexOptions=Index vector (dialog)  Indices=[3]  OutputSizes=1
  Selector2 : Selector  InputPortWidth=4  IndexOptions=Index vector (dialog)  Indices=[4]  OutputSizes=1
  Sum : Sum  Inputs=|++
  Out1 : Outport
  wires:
  Constant/1 -> Sum/2
  In1/1 -> Selector1/1, Selector/1
  In2/1 -> Selector2/1
  Selector1/1 -> Gain1/1
  Mux1/1 -> Out1/1
  Selector2/1 -> Sum/1
  Gain1/1 -> Mux1/2
  Sum/1 -> Mux1/3
  Selector/1 -> Mux1/1

== system MOBATSim/Vehicle Model 3/Longitudinal Speed Control ==
  note: Here the measured speed and the actual speed are the same
      | but it is designed to include the effects of the measurement errors
  note: The vehicle calculates the speed difference between the actual speed and the reference speed, then generates the acceleration command accordingly.
  Speed Reference : Inport
  Inter Vehicular Distance : Inport  Port=2
  Lead Speed : Inport  Port=3
  Driving Mode : Inport  Port=4
  Dist2Stop : Inport  Port=5
  Acceleration Command : Subsystem
  Distance to Stop Controller : Subsystem
  Platoon Controller : Subsystem
  Reference speed according to the driving mode : Subsystem
  Signal Specification1 : SignalSpecification  Dimensions=1
  Sum13 : Sum  Inputs=|+-
  Vehicle Dynamic Model : Subsystem
  Actual Speed : Outport  VectorParamsAs1DForOutWhenUnconnected=off
  Measured Speed : Outport  Port=2  VectorParamsAs1DForOutWhenUnconnected=off
  wires:
  Platoon Controller/1(ref speed) -> Distance to Stop Controller/1(Speed Ref from Platoon), Reference speed according to the driving mode/3(In3)
  Lead Speed/1 -> Platoon Controller/2(Lead Speed)
  Driving Mode/1 -> Acceleration Command/1(Driving Mode), Reference speed according to the driving mode/1(In1)
  Signal Specification1/1 -> Actual Speed/1
  Sum13/1 -> Acceleration Command/2(Speed Error)
  Inter Vehicular Distance/1 -> Platoon Controller/1(Inter Vehicular Distance)
  Dist2Stop/1 -> Distance to Stop Controller/2(Distance to Stop)
  Speed Reference/1 -> Reference speed according to the driving mode/2(In2)
  Distance to Stop Controller/1(ref speed) -> Reference speed according to the driving mode/4(In4)
  Reference speed according to the driving mode/1(Out1) -> Sum13/1
  Vehicle Dynamic Model/1(Vehicle Speed) -> Signal Specification1/1, Acceleration Command/3(Actual Speed), Sum13/2, Platoon Controller/3(Vehicle Speed), Measured Speed/1
  Acceleration Command/1(Acceleration Command) -> Vehicle Dynamic Model/1(Acceleration Command)

== system MOBATSim/Vehicle Model 4/Longitudinal Speed Control ==
  note: Here the measured speed and the actual speed are the same
      | but it is designed to include the effects of the measurement errors
  note: The vehicle calculates the speed difference between the actual speed and the reference speed, then generates the acceleration command accordingly.
  Speed Reference : Inport
  Inter Vehicular Distance : Inport  Port=2
  Lead Speed : Inport  Port=3
  Driving Mode : Inport  Port=4
  Dist2Stop : Inport  Port=5
  Acceleration Command : Subsystem
  Distance to Stop Controller : Subsystem
  Platoon Controller : Subsystem
  Reference speed according to the driving mode : Subsystem
  Signal Specification1 : SignalSpecification  Dimensions=1
  Sum13 : Sum  Inputs=|+-
  Vehicle Dynamic Model : Subsystem
  Actual Speed : Outport  VectorParamsAs1DForOutWhenUnconnected=off
  Measured Speed : Outport  Port=2  VectorParamsAs1DForOutWhenUnconnected=off
  wires:
  Platoon Controller/1(ref speed) -> Distance to Stop Controller/1(Speed Ref from Platoon), Reference speed according to the driving mode/3(In3)
  Lead Speed/1 -> Platoon Controller/2(Lead Speed)
  Driving Mode/1 -> Acceleration Command/1(Driving Mode), Reference speed according to the driving mode/1(In1)
  Signal Specification1/1 -> Actual Speed/1
  Sum13/1 -> Acceleration Command/2(Speed Error)
  Inter Vehicular Distance/1 -> Platoon Controller/1(Inter Vehicular Distance)
  Dist2Stop/1 -> Distance to Stop Controller/2(Distance to Stop)
  Speed Reference/1 -> Reference speed according to the driving mode/2(In2)
  Distance to Stop Controller/1(ref speed) -> Reference speed according to the driving mode/4(In4)
  Reference speed according to the driving mode/1(Out1) -> Sum13/1
  Vehicle Dynamic Model/1(Vehicle Speed) -> Signal Specification1/1, Acceleration Command/3(Actual Speed), Sum13/2, Platoon Controller/3(Vehicle Speed), Measured Speed/1
  Acceleration Command/1(Acceleration Command) -> Vehicle Dynamic Model/1(Acceleration Command)

== system MOBATSim/Vehicle Model 5/Longitudinal Speed Control ==
  note: Here the measured speed and the actual speed are the same
      | but it is designed to include the effects of the measurement errors
  note: The vehicle calculates the speed difference between the actual speed and the reference speed, then generates the acceleration command accordingly.
  Speed Reference : Inport
  Inter Vehicular Distance : Inport  Port=2
  Lead Speed : Inport  Port=3
  Driving Mode : Inport  Port=4
  Dist2Stop : Inport  Port=5
  Acceleration Command : Subsystem
  Distance to Stop Controller : Subsystem
  Platoon Controller : Subsystem
  Reference speed according to the driving mode : Subsystem
  Signal Specification1 : SignalSpecification  Dimensions=1
  Sum13 : Sum  Inputs=|+-
  Vehicle Dynamic Model : Subsystem
  Actual Speed : Outport  VectorParamsAs1DForOutWhenUnconnected=off
  Measured Speed : Outport  Port=2  VectorParamsAs1DForOutWhenUnconnected=off
  wires:
  Platoon Controller/1(ref speed) -> Distance to Stop Controller/1(Speed Ref from Platoon), Reference speed according to the driving mode/3(In3)
  Lead Speed/1 -> Platoon Controller/2(Lead Speed)
  Driving Mode/1 -> Acceleration Command/1(Driving Mode), Reference speed according to the driving mode/1(In1)
  Signal Specification1/1 -> Actual Speed/1
  Sum13/1 -> Acceleration Command/2(Speed Error)
  Inter Vehicular Distance/1 -> Platoon Controller/1(Inter Vehicular Distance)
  Dist2Stop/1 -> Distance to Stop Controller/2(Distance to Stop)
  Speed Reference/1 -> Reference speed according to the driving mode/2(In2)
  Distance to Stop Controller/1(ref speed) -> Reference speed according to the driving mode/4(In4)
  Reference speed according to the driving mode/1(Out1) -> Sum13/1
  Vehicle Dynamic Model/1(Vehicle Speed) -> Signal Specification1/1, Acceleration Command/3(Actual Speed), Sum13/2, Platoon Controller/3(Vehicle Speed), Measured Speed/1
  Acceleration Command/1(Acceleration Command) -> Vehicle Dynamic Model/1(Acceleration Command)

== system MOBATSim/Vehicle Model 6/Longitudinal Speed Control ==
  note: Here the measured speed and the actual speed are the same
      | but it is designed to include the effects of the measurement errors
  note: The vehicle calculates the speed difference between the actual speed and the reference speed, then generates the acceleration command accordingly.
  Speed Reference : Inport
  Inter Vehicular Distance : Inport  Port=2
  Lead Speed : Inport  Port=3
  Driving Mode : Inport  Port=4
  Dist2Stop : Inport  Port=5
  Acceleration Command : Subsystem
  Distance to Stop Controller : Subsystem
  Platoon Controller : Subsystem
  Reference speed according to the driving mode : Subsystem
  Signal Specification1 : SignalSpecification  Dimensions=1
  Sum13 : Sum  Inputs=|+-
  Vehicle Dynamic Model : Subsystem
  Actual Speed : Outport  VectorParamsAs1DForOutWhenUnconnected=off
  Measured Speed : Outport  Port=2  VectorParamsAs1DForOutWhenUnconnected=off
  wires:
  Platoon Controller/1(ref speed) -> Distance to Stop Controller/1(Speed Ref from Platoon), Reference speed according to the driving mode/3(In3)
  Lead Speed/1 -> Platoon Controller/2(Lead Speed)
  Driving Mode/1 -> Acceleration Command/1(Driving Mode), Reference speed according to the driving mode/1(In1)
  Signal Specification1/1 -> Actual Speed/1
  Sum13/1 -> Acceleration Command/2(Speed Error)
  Inter Vehicular Distance/1 -> Platoon Controller/1(Inter Vehicular Distance)
  Dist2Stop/1 -> Distance to Stop Controller/2(Distance to Stop)
  Speed Reference/1 -> Reference speed according to the driving mode/2(In2)
  Distance to Stop Controller/1(ref speed) -> Reference speed according to the driving mode/4(In4)
  Reference speed according to the driving mode/1(Out1) -> Sum13/1
  Vehicle Dynamic Model/1(Vehicle Speed) -> Signal Specification1/1, Acceleration Command/3(Actual Speed), Sum13/2, Platoon Controller/3(Vehicle Speed), Measured Speed/1
  Acceleration Command/1(Acceleration Command) -> Vehicle Dynamic Model/1(Acceleration Command)

== system MOBATSim/Vehicle Model 7/Longitudinal Speed Control ==
  note: Here the measured speed and the actual speed are the same
      | but it is designed to include the effects of the measurement errors
  note: The vehicle calculates the speed difference between the actual speed and the reference speed, then generates the acceleration command accordingly.
  Speed Reference : Inport
  Inter Vehicular Distance : Inport  Port=2
  Lead Speed : Inport  Port=3
  Driving Mode : Inport  Port=4
  Dist2Stop : Inport  Port=5
  Acceleration Command : Subsystem
  Distance to Stop Controller : Subsystem
  Platoon Controller : Subsystem
  Reference speed according to the driving mode : Subsystem
  Signal Specification1 : SignalSpecification  Dimensions=1
  Sum13 : Sum  Inputs=|+-
  Vehicle Dynamic Model : Subsystem
  Actual Speed : Outport  VectorParamsAs1DForOutWhenUnconnected=off
  Measured Speed : Outport  Port=2  VectorParamsAs1DForOutWhenUnconnected=off
  wires:
  Platoon Controller/1(ref speed) -> Distance to Stop Controller/1(Speed Ref from Platoon), Reference speed according to the driving mode/3(In3)
  Lead Speed/1 -> Platoon Controller/2(Lead Speed)
  Driving Mode/1 -> Acceleration Command/1(Driving Mode), Reference speed according to the driving mode/1(In1)
  Signal Specification1/1 -> Actual Speed/1
  Sum13/1 -> Acceleration Command/2(Speed Error)
  Inter Vehicular Distance/1 -> Platoon Controller/1(Inter Vehicular Distance)
  Dist2Stop/1 -> Distance to Stop Controller/2(Distance to Stop)
  Speed Reference/1 -> Reference speed according to the driving mode/2(In2)
  Distance to Stop Controller/1(ref speed) -> Reference speed according to the driving mode/4(In4)
  Reference speed according to the driving mode/1(Out1) -> Sum13/1
  Vehicle Dynamic Model/1(Vehicle Speed) -> Signal Specification1/1, Acceleration Command/3(Actual Speed), Sum13/2, Platoon Controller/3(Vehicle Speed), Measured Speed/1
  Acceleration Command/1(Acceleration Command) -> Vehicle Dynamic Model/1(Acceleration Command)

== system MOBATSim/Vehicle Model 8/Longitudinal Speed Control ==
  note: Here the measured speed and the actual speed are the same
      | but it is designed to include the effects of the measurement errors
  note: The vehicle calculates the speed difference between the actual speed and the reference speed, then generates the acceleration command accordingly.
  Speed Reference : Inport
  Inter Vehicular Distance : Inport  Port=2
  Lead Speed : Inport  Port=3
  Driving Mode : Inport  Port=4
  Dist2Stop : Inport  Port=5
  Acceleration Command : Subsystem
  Distance to Stop Controller : Subsystem
  Platoon Controller : Subsystem
  Reference speed according to the driving mode : Subsystem
  Signal Specification1 : SignalSpecification  Dimensions=1
  Sum13 : Sum  Inputs=|+-
  Vehicle Dynamic Model : Subsystem
  Actual Speed : Outport  VectorParamsAs1DForOutWhenUnconnected=off
  Measured Speed : Outport  Port=2  VectorParamsAs1DForOutWhenUnconnected=off
  wires:
  Platoon Controller/1(ref speed) -> Distance to Stop Controller/1(Speed Ref from Platoon), Reference speed according to the driving mode/3(In3)
  Lead Speed/1 -> Platoon Controller/2(Lead Speed)
  Driving Mode/1 -> Acceleration Command/1(Driving Mode), Reference speed according to the driving mode/1(In1)
  Signal Specification1/1 -> Actual Speed/1
  Sum13/1 -> Acceleration Command/2(Speed Error)
  Inter Vehicular Distance/1 -> Platoon Controller/1(Inter Vehicular Distance)
  Dist2Stop/1 -> Distance to Stop Controller/2(Distance to Stop)
  Speed Reference/1 -> Reference speed according to the driving mode/2(In2)
  Distance to Stop Controller/1(ref speed) -> Reference speed according to the driving mode/4(In4)
  Reference speed according to the driving mode/1(Out1) -> Sum13/1
  Vehicle Dynamic Model/1(Vehicle Speed) -> Signal Specification1/1, Acceleration Command/3(Actual Speed), Sum13/2, Platoon Controller/3(Vehicle Speed), Measured Speed/1
  Acceleration Command/1(Acceleration Command) -> Vehicle Dynamic Model/1(Acceleration Command)
